simulink model "untitled"  (Simulink 7.7)
settings: Solver=ode45  StartTime=0.0  StopTime=10.0  RelTol=1e-3
settings Model: Creator=alexey  LastModifiedBy=alexey

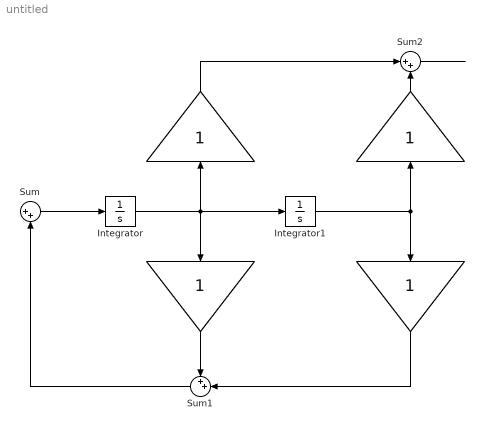
== system untitled ==
  " " : Gain
  "  " : Gain
  "     " : Gain
  "      " : Gain
  Integrator : Integrator
  Integrator1 : Integrator
  Sum : Sum  Inputs=|++
  Sum1 : Sum  Inputs=++|
  Sum2 : Sum  Inputs=|++
  wires:
  Sum/1 -> Integrator/1
  Integrator/1 -> Integrator1/1, "  "/1, "     "/1
  "  "/1 -> Sum1/1
  " "/1 -> Sum1/2
  Integrator1/1 -> "      "/1, " "/1
  "     "/1 -> Sum2/1
  "      "/1 -> Sum2/2
  Sum1/1 -> Sum/2
  ? -> Sum/1
  Sum2/1 -> ?
